simulink model "lightcontrol_ifelse"  (R2020a)
settings: Solver=FixedStepAuto  StartTime=0.0  StopTime=20  FixedStep=0.01  RelTol=1e-3
undefined symbols (not defined in the file): sigbuilder_block
settings Model: Creator=shushushu  LastModifiedBy=shushushu

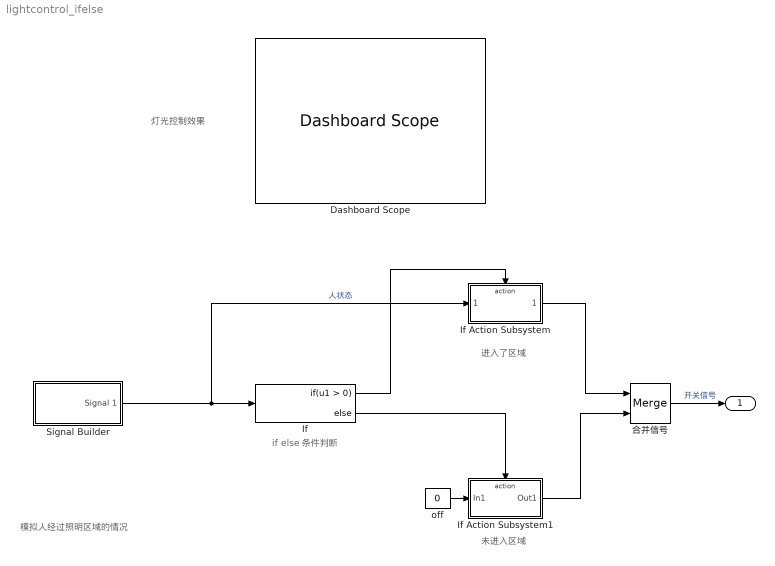
== system lightcontrol_ifelse ==
  note: 灯光控制效果
  note: 模拟人经过照明区域的情况
  note: 进入了区域
  note: 未进入区域
  note: if else 条件判断
  Dashboard Scope : DashboardScope  Ymin=0  Ymax=1
  If : If
  If Action Subsystem : Subsystem  TreatAsAtomicUnit=on
  If Action Subsystem1 : Subsystem  TreatAsAtomicUnit=on
  Signal Builder : Subsystem  Tag=STV Subsys  LoadFcn=sigbuilder_block('load');  StartFcn=sigbuilder_block('start');  StopFcn=sigbuilder_block('stop');  ClipboardFcn=sigbuilder_block('clipboard');  mask(Sigbuilder block){tuvar=[0:10]}
      mask help: Simulink:masks:SigbuilderBlock_MD
      mask init:
      | if ~strcmp(get_param(bdroot(gcbh),'SimulationStatus'),'stopped') tuvar = sigbuilder_block('maskInit'); end
      settings: CopyFcn=sigbuilder_block('copy');  DeleteFcn=sigbuilder_block('delete');  ModelCloseFcn=sigbuilder_block('modelClose');  PreSaveFcn=sigbuilder_block('preSave');  PauseFcn=sigbuilder_block('pause');  ContinueFcn=sigbuilder_block('continue');  NameChangeFcn=sigbuilder_block('namechange');  OpenFcn=sigbuilder_block('open',[542.25 217.5 550.5 358.5 ]);  CloseFcn=sigbuilder_block('close');
      mask Display: plot(0, 0, 100, 100,[2, 2, 32, 32, 2], [68, 8, 8, 68, 68],[32, 2], [38, 38], [32, 19, 2],[53, 60, 44], [32, 17, 17, 2],[16, 16, 31, 31]);txt = getActiveGroup(gcbh);text(2, 100, txt,'verticalAlignment', 'top');
  off : Constant  Value=0  VectorParams1D=off  SampleTime=-1
  合并信号 : Merge
  " " : Outport
  wires:
  If/1 -> If Action Subsystem/Action
  If/2 -> If Action Subsystem1/Action
  off/1 -> If Action Subsystem1/1(In1)
  If Action Subsystem/1(lighton) -> 合并信号/1
  If Action Subsystem1/1(Out1) -> 合并信号/2
  合并信号/1 -> " "/1  "开关信号"
  Signal Builder/1(Signal 1) -> If Action Subsystem/1(peoplein), If/1  "人状态"

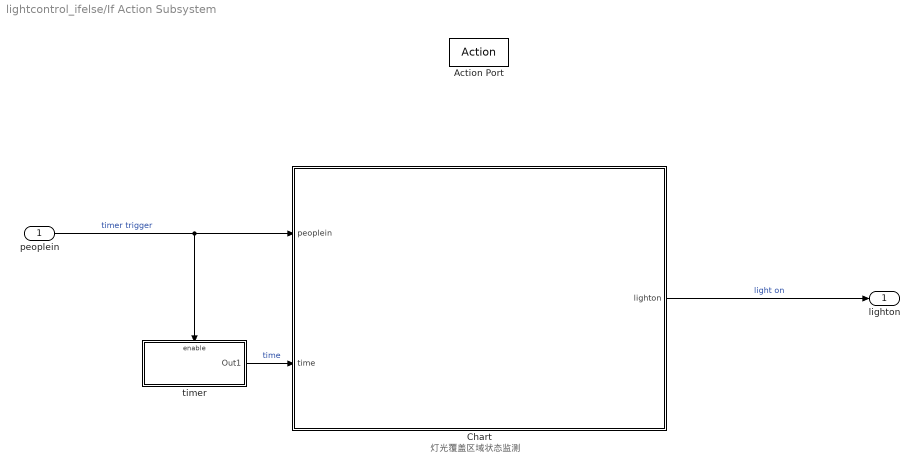
== system lightcontrol_ifelse/If Action Subsystem ==
  note: 灯光覆盖区域状态监测
  peoplein : Inport
  Action Port : ActionPort  InitializeStates=reset  ActionPortLabel=if(u1 > 0)
  Chart : Stateflow chart  TreatAsAtomicUnit=on
  timer : Subsystem
  lighton : Outport
  wires:
  Chart/1(lighton) -> lighton/1  "light on"
  timer/1(Out1) -> Chart/2(time)  "time"
  peoplein/1 -> timer/Enable, Chart/1(peoplein)  "timer trigger"

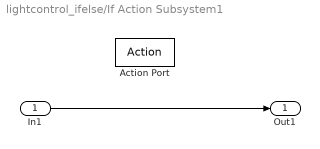
== system lightcontrol_ifelse/If Action Subsystem1 ==
  In1 : Inport
  Action Port : ActionPort  ActionPortLabel=else
  Out1 : Outport
  wires:
  In1/1 -> Out1/1

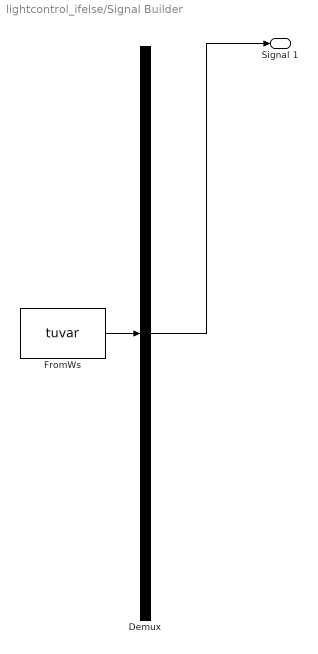
== system lightcontrol_ifelse/Signal Builder ==
  Demux : Demux  Tag=STV Demux  Outputs=1
      settings: DisplayOption=none
  FromWs : FromWorkspace  Tag=STV FromWs  VariableName=tuvar
      SigBuilderData=|
      | common.afterFinalStr = 'Extrapolate'
      | common.sampleTime = 0
      | dataSet.timeRange = [0 10]
      | dataSet.name = 'Group 1'
      | sbobj.Groups.Name = 'Group 1'
      | sbobj.Groups.Signals.Name = 'Signal 1'
      | sbobj.Groups.Signals.XData = [0 0.98 0.98 8 8 10]
      | sbobj.Groups.Signals.YData = [0 0 1.035 1.035 0 0]
  Signal 1 : Outport  Tag=STV Outport
  wires:
  Demux/1 -> Signal 1/1
  FromWs/1 -> Demux/1

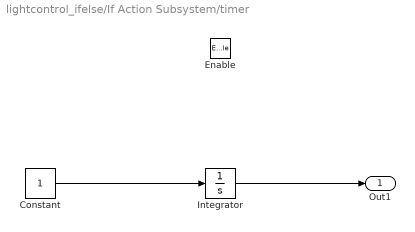
== system lightcontrol_ifelse/If Action Subsystem/timer ==
  Enable : EnablePort
  Constant : Constant
  Integrator : Integrator
  Out1 : Outport
  wires:
  Constant/1 -> Integrator/1
  Integrator/1 -> Out1/1

== stateflow chart lightcontrol_ifelse/If Action Subsystem/Chart ==
  state Leave_area
    en:lighton = 1;
  state In_area
    en:lighton = 0;
  (default) -> In_area
  In_area -> Leave_area : [[peoplein > 0] & [ time >= 3]]
  Leave_area -> In_area : [peoplein==0]
  data: peoplein input; time input; lighton output
